simulink model "hmiTest"  (R2017a)
settings: Solver=FixedStepAuto  StartTime=0.0  StopTime=inf  RelTol=1e-3
undefined symbols (not defined in the file): vrrotmat2vec
libraries: vrlib x3, myo_lib x3, aerolibconvert2 x2, dspstat3 x2, sldrtlib x1
settings Model: Creator=ricardog  LastModifiedBy=ricardog
settings SolverCC: AutoInsertRateTranBlk=on

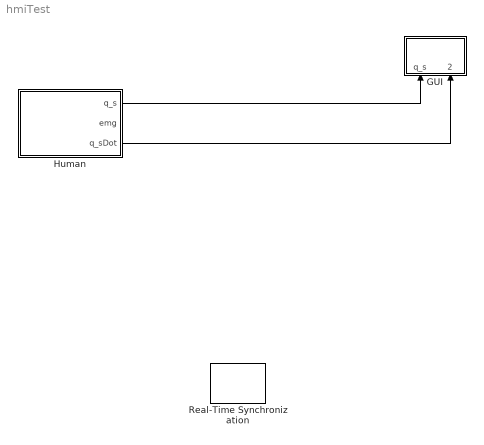
== system hmiTest ==
  GUI : Subsystem
  Human : Subsystem
  Real-Time Synchronization : sldrtlib/Real-Time Synchronization  SampleTime=0.01  MaxMissedTicks=50  ShowMissedTicks=off  YieldWhenWaiting=off
  wires:
  Human/1(q_s) -> GUI/1(q_s)
  Human/3(q_sDot) -> GUI/2(q_sDot)

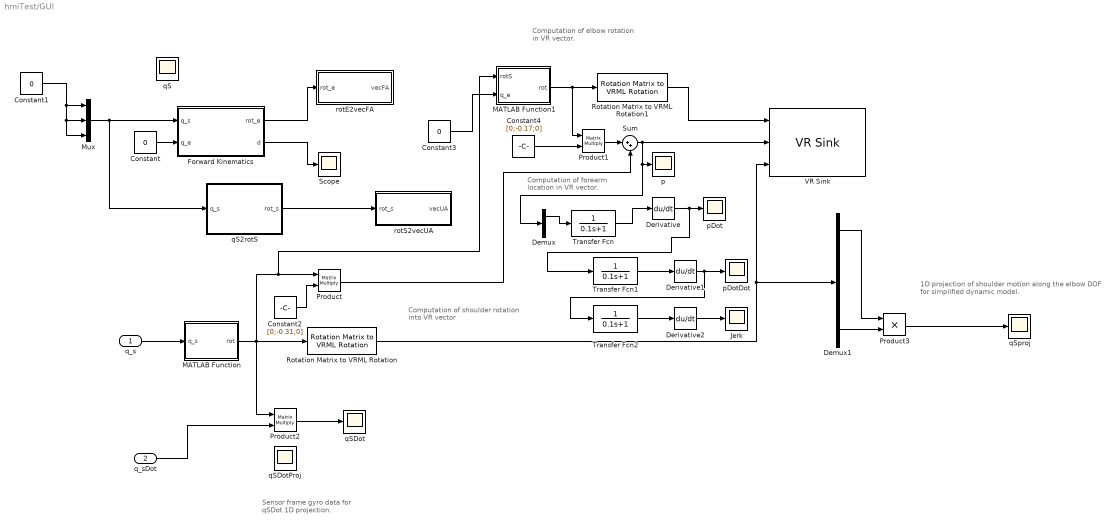
== system hmiTest/GUI ==
  note: Sensor frame gyro data for
      | qSDot 1D projection.
  note: Computation of forearm
      | location in VR vector.
  note: Computation of elbow rotation
      | in VR vector.
  note: Computation of shoulder rotation
      | into VR vector
  note: 1D projection of shoulder motion
      | along the elbow DOF for simplified dynamic model.
  q_s : Inport
  q_sDot : Inport  Port=2
  Constant : Constant  Value=0
  Constant1 : Constant  Value=0
  Constant2 : Constant  Value=[0;-0.31;0]  VectorParams1D=off
  Constant3 : Constant  Value=0
  Constant4 : Constant  Value=[0;-0.17;0]  VectorParams1D=off
  Demux : Demux  Outputs=3
  Demux1 : Demux
  Derivative : Derivative
  Derivative1 : Derivative
  Derivative2 : Derivative
  Forward Kinematics : MATLAB Function  TreatAsAtomicUnit=on
  Jerk : Scope
  MATLAB Function : MATLAB Function  TreatAsAtomicUnit=on
  MATLAB Function1 : MATLAB Function  TreatAsAtomicUnit=on
  Mux : Mux  Inputs=3
  Product : Product  Multiplication=Matrix(*)
  Product1 : Product  Multiplication=Matrix(*)
  Product2 : Product  Multiplication=Matrix(*)
  Product3 : Product
  Rotation Matrix to VRML Rotation : vrlib/Utilities/Rotation Matrix to VRML Rotation  maxzero=1e-12
      settings: SourceProductName=Simulink 3D Animation  SourceProductBaseCode=VR
  Rotation Matrix to VRML Rotation1 : vrlib/Utilities/Rotation Matrix to VRML Rotation  maxzero=1e-12
      settings: SourceProductName=Simulink 3D Animation  SourceProductBaseCode=VR
  Scope : Scope
  Sum : Sum  Inputs=|++
  Transfer Fcn : TransferFcn  Denominator=[0.1 1]
  Transfer Fcn1 : TransferFcn  Denominator=[0.1 1]
  Transfer Fcn2 : TransferFcn  Denominator=[0.1 1]
  VR Sink : vrlib/VR Sink  InstantiateOnLoad=on  SampleTime=0.1  ViewEnable=on  RemoteChange=off  RemoteView=off  FieldsWritten=Forearm.rotation.4.1.1.double#Forearm.translation.3.1.1.double#UpperArm.rotation.4.1.1.double  WorldFileName=C:\Users\ricardog\Documents\Workspace\IterativeSynergyLearning\GUI\VR\armTargetsVR.wrl  AutoView=on  VideoDimensions=[]  AllowVariableSize=off  FigureProperties="{'Position', 'Name', 'Viewpoint', 'CameraBound', 'CameraDirection', 'CameraPosition', 'CameraUpVector', 'ZoomFactor', 'Antialiasing', 'Headlight', 'Lighting', 'NavPanel', 'Sound', 'StatusBar', 'Stereo3D', 'Stereo3DCameraOffset', 'Stereo3DHIT', 'ToolBar', 'Textures', 'Transparency', 'Triad', 'Wireframe', 'NavZones', 'NavMode', 'NavSpeed', 'CaptureFileFormat', 'CaptureFileName', 'Record2DCompressMethod', 'Record2DCompressQuality', 'Record2D', 'Record2DFileName', 'Record2DFPS'; [1.7986000000000001e+03   1.8779999999999995e+02   5.7600000000000000e+02   3.7000000000000000e+02], '', 'FPV', 'on', [0.0000000000000000e+00   0.0000000000000000e+00  -1.0000000000000000e+00], [0.0000000000000000e+00   0.0000000000000000e+00   0.0000000000000000e+00], [0.0000000000000000e+00   1.0000000000000000e+00   0.0000000000000000e+00], [1.0000000000000000e+00], 'on', 'on', 'on', 'halfbar', 'on', 'on', 'off', [1.0000000149011612e-01], [0.0000000000000000e+00], 'on', 'on', 'on', 'none', 'off', 'off', 'fly', 'normal', 'tif', '%f_anim_%n.tif', 'auto', [7.5000000000000000e+01], 'off', '%f_anim_%n.avi', 'auto'}"
      settings: SourceProductBaseCode=VR
  p : Scope
  pDot : Scope
  pDotDot : Scope
  qS : Scope
  qS2rotS : MATLAB Function  TreatAsAtomicUnit=on
  qSDot : Scope
  qSDotProj : Scope
  qSproj : Scope
  rotE2vecFA : Subsystem
  rotS2vecUA : Subsystem
  wires:
  Forward Kinematics/2(d) -> Scope/1
  Forward Kinematics/1(rot_e) -> rotE2vecFA/1(rot_e)
  qS2rotS/1(rot_s) -> rotS2vecUA/1(rot_s)
  Constant/1 -> Forward Kinematics/2(q_e)
  Mux/1 -> qS2rotS/1(q_s), Forward Kinematics/1(q_s)
  Constant1/1 -> Mux/1, Mux/2, Mux/3
  q_s/1 -> MATLAB Function/1(q_s)
  MATLAB Function/1(rot) -> Product2/1, MATLAB Function1/1(rotS), Product/1, Rotation Matrix to VRML Rotation/1
  Constant2/1 -> Product/2
  Constant3/1 -> MATLAB Function1/2(q_e)
  MATLAB Function1/1(rot) -> Product1/1, Rotation Matrix to VRML Rotation1/1
  Rotation Matrix to VRML Rotation1/1 -> VR Sink/1
  Constant4/1 -> Product1/2
  Product1/1 -> Sum/1
  Product/1 -> Sum/2
  Sum/1 -> VR Sink/2, Demux/1, p/1
  Rotation Matrix to VRML Rotation/1 -> VR Sink/3, Demux1/1
  Demux1/4 -> Product3/2
  Product3/1 -> qSproj/1
  Demux1/1 -> Product3/1
  Product2/1 -> qSDot/1
  q_sDot/1 -> Product2/2
  Derivative1/1 -> Transfer Fcn2/1, pDotDot/1
  Derivative2/1 -> Jerk/1
  Transfer Fcn/1 -> Derivative/1
  Demux/1 -> Transfer Fcn/1
  Transfer Fcn1/1 -> Derivative1/1
  Derivative/1 -> Transfer Fcn1/1, pDot/1
  Transfer Fcn2/1 -> Derivative2/1

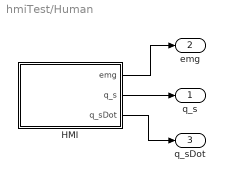
== system hmiTest/Human ==
  HMI : Subsystem
  q_s : Outport
  emg : Outport  Port=2
  q_sDot : Outport  Port=3
  wires:
  HMI/1(emg) -> emg/1
  HMI/2(q_s) -> q_s/1
  HMI/3(q_sDot) -> q_sDot/1

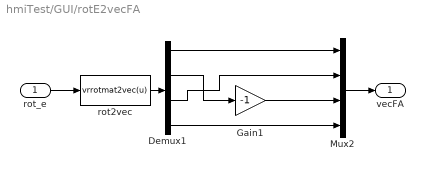
== system hmiTest/GUI/rotE2vecFA ==
  rot_e : Inport
  Demux1 : Demux
  Gain1 : Gain  Gain=-1
  Mux2 : Mux
  rot2vec : MATLABFcn  MATLABFcn=vrrotmat2vec(u)
  vecFA : Outport
  wires:
  Demux1/3 -> Mux2/2
  Demux1/4 -> Mux2/4
  rot2vec/1 -> Demux1/1
  Demux1/1 -> Mux2/1
  Gain1/1 -> Mux2/3
  Demux1/2 -> Gain1/1
  Mux2/1 -> vecFA/1
  rot_e/1 -> rot2vec/1

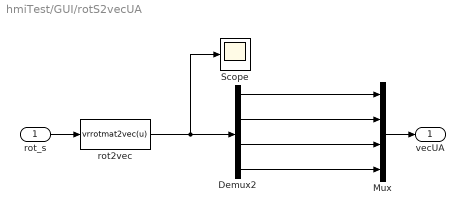
== system hmiTest/GUI/rotS2vecUA ==
  rot_s : Inport
  Demux2 : Demux
  Mux : Mux
  Scope : Scope
  rot2vec : MATLABFcn  MATLABFcn=vrrotmat2vec(u)
  vecUA : Outport
  wires:
  Demux2/1 -> Mux/1
  Demux2/4 -> Mux/4
  rot2vec/1 -> Scope/1, Demux2/1
  Mux/1 -> vecUA/1
  rot_s/1 -> rot2vec/1
  Demux2/2 -> Mux/2
  Demux2/3 -> Mux/3

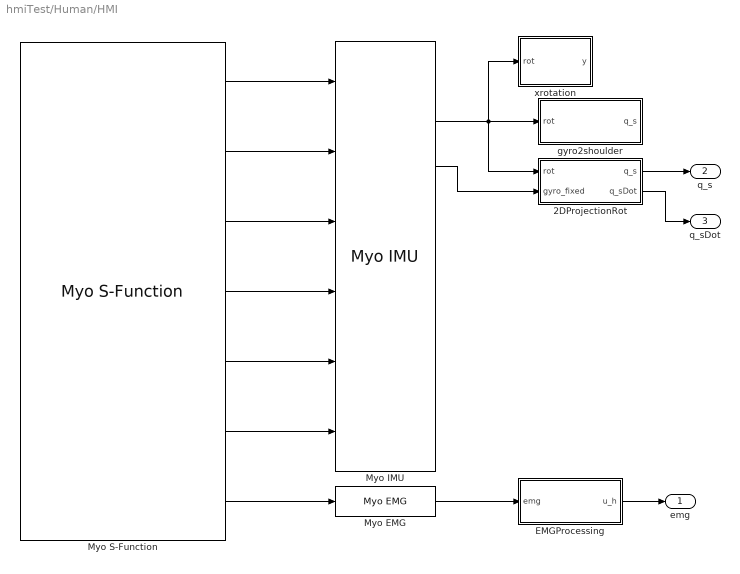
== system hmiTest/Human/HMI ==
  2DProjectionRot : Subsystem
  EMGProcessing : Subsystem
  Myo EMG : myo_lib/Myo EMG
  Myo IMU : myo_lib/Myo IMU
  Myo S-Function : myo_lib/Myo S-Function  emgEnabled=1  countMyos=1
  gyro2shoulder : Subsystem
  xrotation : MATLAB Function  TreatAsAtomicUnit=on
  emg : Outport
  q_s : Outport  Port=2
  q_sDot : Outport  Port=3
  wires:
  Myo S-Function/3 -> Myo IMU/3
  Myo S-Function/7 -> Myo EMG/1
  Myo S-Function/4 -> Myo IMU/4
  Myo S-Function/5 -> Myo IMU/5
  Myo S-Function/2 -> Myo IMU/2
  Myo S-Function/1 -> Myo IMU/1
  Myo S-Function/6 -> Myo IMU/6
  Myo EMG/1 -> EMGProcessing/1(emg)
  EMGProcessing/1(u_h) -> emg/1
  Myo IMU/2 -> xrotation/1(rot), gyro2shoulder/1(rot), 2DProjectionRot/1(rot)
  2DProjectionRot/1(q_s) -> q_s/1
  2DProjectionRot/2(q_sDot) -> q_sDot/1
  Myo IMU/3 -> 2DProjectionRot/2(gyro_fixed)

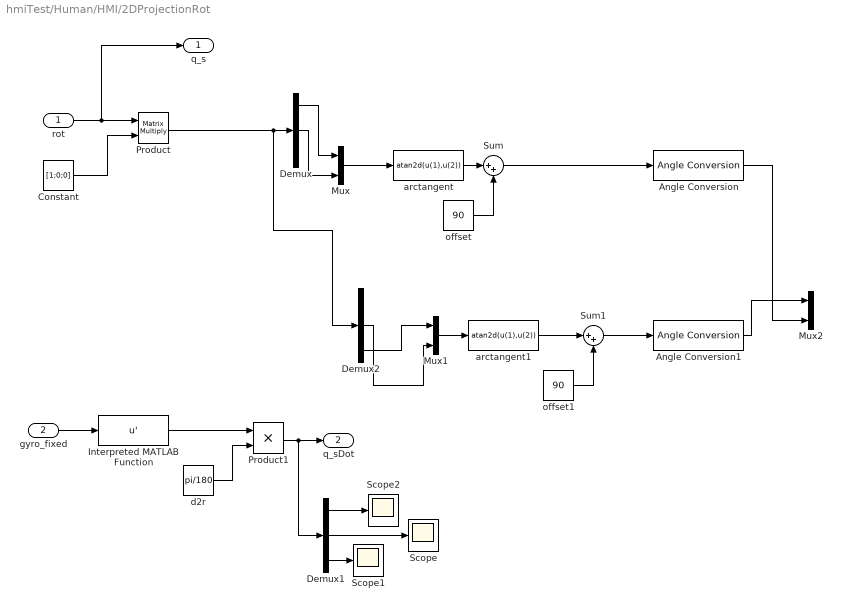
== system hmiTest/Human/HMI/2DProjectionRot ==
  rot : Inport
  gyro_fixed : Inport  Port=2
  Angle Conversion : aerolibconvert2/Angle Conversion  IU=deg  OU=rad
  Angle Conversion1 : aerolibconvert2/Angle Conversion  IU=deg  OU=rad
  Constant : Constant  Value=[1;0;0]  VectorParams1D=off
  Demux : Demux  Outputs=3
  Demux1 : Demux  Outputs=3
  Demux2 : Demux  Outputs=3
  Interpreted MATLAB Function : MATLABFcn  MATLABFcn=u'
  Mux : Mux  Inputs=2
  Mux1 : Mux  Inputs=2
  Mux2 : Mux  Inputs=2
  Product : Product  Multiplication=Matrix(*)
  Product1 : Product
  Scope : Scope
  Scope1 : Scope
  Scope2 : Scope
  Sum : Sum  Inputs=|++
  Sum1 : Sum  Inputs=|++
  arctangent : MATLABFcn  MATLABFcn=atan2d(u(1),u(2))
  arctangent1 : MATLABFcn  MATLABFcn=atan2d(u(1),u(2))
  d2r : Constant  Value=pi/180
  offset : Constant  Value=90
  offset1 : Constant  Value=90
  q_s : Outport
  q_sDot : Outport  Port=2
  wires:
  rot/1 -> q_s/1, Product/1
  Constant/1 -> Product/2
  Product/1 -> Demux2/1, Demux/1
  arctangent/1 -> Sum/1
  offset/1 -> Sum/2
  Sum/1 -> Angle Conversion/1
  d2r/1 -> Product1/2
  Angle Conversion1/1 -> Mux2/1
  Angle Conversion/1 -> Mux2/2
  Demux2/3 -> Mux1/1
  offset1/1 -> Sum1/2
  arctangent1/1 -> Sum1/1
  Sum1/1 -> Angle Conversion1/1
  Mux/1 -> arctangent/1
  Mux1/1 -> arctangent1/1
  Demux2/2 -> Mux1/2
  Demux/1 -> Mux/1
  Demux/2 -> Mux/2
  Product1/1 -> Demux1/1, q_sDot/1
  gyro_fixed/1 -> Interpreted MATLAB Function/1
  Interpreted MATLAB Function/1 -> Product1/1
  Demux1/3 -> Scope1/1
  Demux1/2 -> Scope/1
  Demux1/1 -> Scope2/1

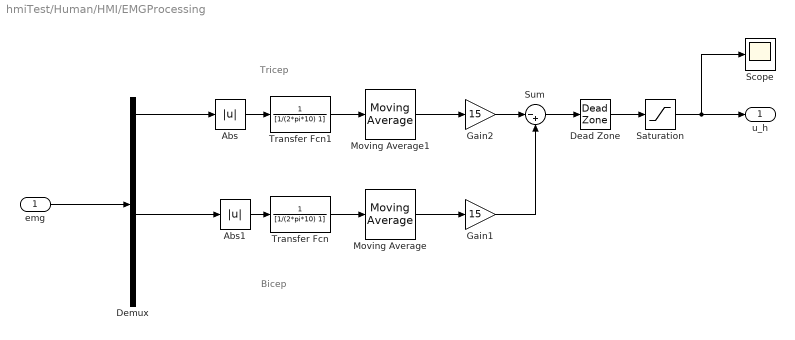
== system hmiTest/Human/HMI/EMGProcessing ==
  note: Tricep
  note: Bicep
  emg : Inport
  Abs : Abs
  Abs1 : Abs
  Dead Zone : DeadZone  SaturateOnIntegerOverflow=on
  Demux : Demux  Outputs=8
  Gain1 : Gain  Gain=15
  Gain2 : Gain  Gain=15
  Moving Average : dspstat3/Moving Average  Method=Sliding window  SpecifyWindowLength=on  WindowLength=1000  ForgettingFactor=0.9  SimulateUsing=Code generation
  Moving Average1 : dspstat3/Moving Average  Method=Sliding window  SpecifyWindowLength=on  WindowLength=1000  ForgettingFactor=0.9  SimulateUsing=Code generation
  Saturation : Saturate  UpperLimit=3  LowerLimit=-3
  Scope : Scope
  Sum : Sum  Inputs=|-+
  Transfer Fcn : TransferFcn  Denominator=[1/(2*pi*10) 1]
  Transfer Fcn1 : TransferFcn  Denominator=[1/(2*pi*10) 1]
  u_h : Outport
  wires:
  Transfer Fcn/1 -> Moving Average/1
  Moving Average/1 -> Gain1/1
  Moving Average1/1 -> Gain2/1
  Demux/5 -> Abs1/1
  Demux/1 -> Abs/1
  Abs1/1 -> Transfer Fcn/1
  Transfer Fcn1/1 -> Moving Average1/1
  Abs/1 -> Transfer Fcn1/1
  emg/1 -> Demux/1
  Gain1/1 -> Sum/2
  Gain2/1 -> Sum/1
  Saturation/1 -> Scope/1, u_h/1
  Sum/1 -> Dead Zone/1
  Dead Zone/1 -> Saturation/1

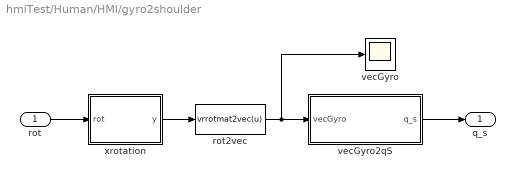
== system hmiTest/Human/HMI/gyro2shoulder ==
  rot : Inport
  rot2vec : MATLABFcn  MATLABFcn=vrrotmat2vec(u)
  vecGyro : Scope
  vecGyro2qS : MATLAB Function  TreatAsAtomicUnit=on
  xrotation : MATLAB Function  TreatAsAtomicUnit=on
  q_s : Outport
  wires:
  rot2vec/1 -> vecGyro2qS/1(vecGyro), vecGyro/1
  vecGyro2qS/1(q_s) -> q_s/1
  xrotation/1(y) -> rot2vec/1
  rot/1 -> xrotation/1(rot)

== matlab function hmiTest/GUI/qS2rotS ==
  data: q_s input; rot_s output
% qS2rotS
% Description
% Transforms gyroscope angle vector to manipulator transformation matrix.
% @in q_s Shoulder angle vector.
% @out rot_s Shoulder manipulator rotation matrix.
function rot_s = qS2rotS(q_s)
la = 0.31;
% Shoulder location offset transformation
% mT01 = T(0,0,0,pi/2);
% mT02 = T(pi/2,0,0,0);
% % Shoulder abduction/adduction
mT1 = T(0,0,0,q_s(1));
% % Shoulder flexion/extension
mT2 = T(-pi/2,0,0,q_s(2)-pi/2);
% % Shoulder rotation
% mT3 = T(-pi/2,0,la,q_s(3));
% Forearm COG location
mT_s = mT1*mT2;
rot_s = [mT_s(1,1:3);
       mT_s(2,1:3);
       mT_s(3,1:3)];
% rot_s = rotx(rad2deg(q_s(1)))*roty(rad2deg(q_s(2)))*roty(rad2deg(q_s(3)));

== matlab function hmiTest/GUI/Forward Kinematics ==
  data: rot_e output; q_s input; d output; q_e input
function [rot_e, d] = forwardKine(q_s,q_e)
la = 0.31;
lf = 0.34;
% Shoulder location offset transformation
mT01 = T(0,0,0,-pi/2);
mT02 = T(pi/2,0,0,-pi/2);
% % Shoulder abduction/adduction
mT1 = T(0,0,0,q_s(1));
% % Shoulder flexion/extension
mT2 = T(-pi/2,0,0,q_s(2)-pi/2);
% % Shoulder rotation
mT3 = T(-pi/2,0,la,q_s(3));
% Elbow flexion/extension
mT4 = T(pi/2,0,0,q_e);
% Forarm link
mT5 = T(-pi/2,0,-lf/2,0);
% Forearm COG location
yrot = roty(180);
mTy = [yrot(1,1:3),0;
       yrot(2,1:3),0;
       yrot(3,1:3),0;
       0,0,0,1];
mT_e = mT01*mT02*mT1*mT2*mT3*mTy*mT4*mT5;
d = [mT_e(1,4);mT_e(3,4);mT_e(2,4)];
rot_e = [mT_e(1,1:3);
       mT_e(2,1:3);
       mT_e(3,1:3)];

== matlab function hmiTest/Human/HMI/gyro2shoulder/vecGyro2qS ==
  data: vecGyro input; q_s output
% vecGyro2qS
% Description
% Transforms myoband gyroscope rotation matrix to a three angle vector.
% @in vecGyro Gyroscope angle vector.
% @out q_s shoulder angle vector.
function q_s = vecGyro2qS(vecGyro)
% vecGyro(3): abduction/adduction
% vecGyro(1): rotation
% vecGyro(2): flexion/extension
% q_s = vecGyro(4)*[vecGyro(3);-vecGyro(1);vecGyro(2)]+[0;-pi/2;0];
% q_s = [vecGyro(2);vecGyro(3);vecGyro(1);vecGyro(4)];
% q_s = vecGyro;
q_s = 0;

== matlab function hmiTest/Human/HMI/gyro2shoulder/xrotation ==
  data: rot input; y output
function y = fcn(rot)

% y = rotz(90)*rot;
y = rot;

== matlab function hmiTest/Human/HMI/xrotation ==
  data: rot input; y output
function y = fcn(rot)

y = rot*rotz(90);
% y = rot;

== matlab function hmiTest/GUI/MATLAB Function ==
  data: q_s input; rot output
function rot  = fcn(q_s)
%
% rot = roty(180)*rotx(rad2deg(q_s(1)))*rotz(rad2deg(q_s(2)));
% rot = rotx(rad2deg(q_s(1)))*rotz(rad2deg(q_s(2)));
rot = rotx(-90)*q_s*rotz(90);

== matlab function hmiTest/GUI/MATLAB Function1 ==
  data: rotS input; rot output; q_e input
function rot = fcn(rotS,q_e)
%
% rot = roty(180)*rotx(rad2deg(q_s(1)))*rotz(rad2deg(q_s(2)));
% rot = rotx(rad2deg(q_s(1)))*rotz(rad2deg(q_s(2)));
rot = rotS*rotz(q_e);
